simulink model "temp_ACGen_DCLink"  (R2013b)
settings: Solver=ode3  StartTime=0.0  StopTime=0.7  FixedStep=Ts  RelTol=1e-3
PreLoadFcn:
  | warning off Simulink:Commands:LoadMdlParameterizedLink
  | Ts=1e-5;
PostLoadFcn:
  | warning off Simulink:Commands:LoadMdlParameterizedLink
  | warning off Simulink:Engine:UsingDiscreteSolver
undefined symbols (not defined in the file or in its folder): D1, Delta
libraries: powerlib x21, powerlib_extras x5, Generator_Lib x1, simulink x1
Description:
  | Copyright 2013 The MathWorks, Inc.
settings Model: Creator=smiller  LastModifiedBy=smiller
settings DebuggingCC: StateNameClashWarn=warning

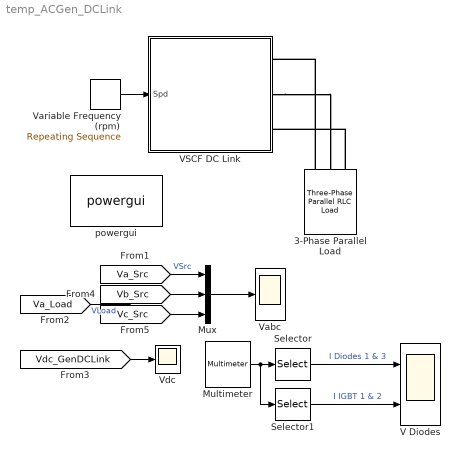
== system temp_ACGen_DCLink ==
  3-Phase Parallel Load : powerlib/Elements/Three-Phase Parallel RLC Load  LConnTagsString=A|B|C  Configuration=Y (grounded)  NominalVoltage=200  NominalFrequency=400  ActivePower=50e3  InductivePower=0  CapacitivePower=0  Measurements=None  LoadType=constant Z
  Multimeter : powerlib/Measurements/Multimeter  Tag=PoWeRsYsTeMmEaSuReMeNt  PhasorSimulation=off  OutputType=Magnitude  sel=[1 3 7 8]  L=12  Gain=[1 1 1 1]  yselected="{'Isw1: VSCF DC Link/Rect and Inv/Rectifier','Isw3: VSCF DC Link/Rect and Inv/Rectifier','Isw1: VSCF DC Link/Rect and Inv/PWM  IGBT Inverter','Isw2: VSCF DC Link/Rect and Inv/PWM  IGBT Inverter'};"  PSBOutputType=1  PSBequivalent=0  AxesSetting=[0,0.1,-100,100]  Display=0  SavedBlockNames=-11
      settings: AttributesFormatString=\n
  Mux : Mux  Inputs=3
  Selector : Selector  InputPortWidth=4  IndexOptions=Index vector (dialog)  Indices=[1 2]  OutputSizes=1
  Selector1 : Selector  InputPortWidth=4  IndexOptions=Index vector (dialog)  Indices=[3 4]  OutputSizes=1
  V Diodes : Scope  NumInputPorts=2
      settings: TimeRange=0.005  YMin=-10~-205  YMax=100~205
  VSCF DC Link : Subsystem
      mask Display:
      | image(imread('Gen_VSCF_DCLink_IMAGE.JPG','jpg'))
      | port_label('RConn',1,'A');
      | port_label('RConn',2,'B');
      | port_label('RConn',3,'C');
      | port_label('Input',1,'Spd');
  Vabc : Scope
      settings: TimeRange=0.0025  YMin=-200  YMax=200
  Variable Frequency (rpm) : simulink/Sources/Repeating Sequence  rep_seq_t=[0 1 2 3 4 5 6 7]/10  rep_seq_y=[1 1 0.9 0.95 0.8 0.96 1 1]*12000
  Vdc : Scope
      settings: TimeRange=0.0025  YMin=780  YMax=790  SaveName=ScopeData2
  powergui : powerlib/powergui  Priority=2  SimulationMode=Discrete  SolverType=Tustin  SampleTime=Ts  frequency=60  SPID=off  DisableSnubberDevices=off  DisableRonSwitches=off  DisableVfSwitches=off  SwTol=0  Interpol=off  DisplayEquations=off  frequencyindice=0  Pbase=100e6  ErrMax=1e-4  Iterations=50  UnitsV=kV  UnitsW=MW  FunctionMessages=off  echomessages=off  HookPort=off  EnableUseOfTLC=off  x0status=blocks  RestoreLinks=warning  ResistiveCurrentMeasurement=off  Frange=[0:2:500]  Ylog=off  Xlog=on  ShowGrid=off  save=off  variable=ZData  structure=psbbridges_str  ZoomFFT=on  StartTime=0.1-2/50  cycles=2  DisplayStyle=off  fundamental=50  FreqAxis=off  MaxFrequency=7000  frequencyindicesteady=1  RmsSteady=1  display=off  Ts=0  methode=off
  wires:
  Variable Frequency (rpm)/1 -> VSCF DC Link/1(Spd)
  [Va_Src] -> Mux/1  "VSrc"
  [Va_Load] -> ?  "VLoad"
  Selector/1 -> V Diodes/1  "I Diodes 1 & 3"
  Selector1/1 -> V Diodes/2  "I IGBT 1 & 2"
  Multimeter/1 -> Selector/1, Selector1/1
  [Vdc_GenDCLink] -> Vdc/1
  Mux/1 -> Vabc/1
  [Vb_Src] -> Mux/2
  [Vc_Src] -> Mux/3
  connections:
  3-Phase Parallel Load/LConn3 -- VSCF DC Link/RConn3
  3-Phase Parallel Load/LConn1 -- VSCF DC Link/RConn1
  VSCF DC Link/RConn2 -- 3-Phase Parallel Load/LConn2

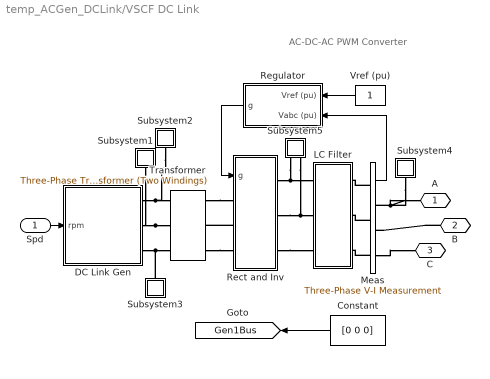
== system temp_ACGen_DCLink/VSCF DC Link ==
  note: AC-DC-AC PWM Converter
  Spd : Inport
  Constant : Constant  Value=[0 0 0]
  DC Link Gen : Subsystem  BlockChoice=Ideal
      settings: AttributesFormatString=%<BlockChoice>  TemplateBlock=Generator_Lib/DC Gen/DC Link Gen  MemberBlocks=Ideal,Sync Mach
  LC Filter : Subsystem
  Meas : powerlib/Measurements/Three-Phase V-I Measurement  VoltageMeasurement=phase-to-ground  SetLabelV=off  LabelV=V1  Vpu=on  VpuLL=off  CurrentMeasurement=no  SetLabelI=off  LabelI=I1  Ipu=off  Pbase=1e3  Vbase=200  OutputType=Magnitude  PhasorSimulation=off  PSBequivalent=0
  Rect and Inv : Subsystem
  Regulator : Subsystem
  Subsystem1 : Subsystem
      mask Display: disp('S')
  Subsystem2 : Subsystem
      mask Display: disp('S')
  Subsystem3 : Subsystem
      mask Display: disp('S')
  Subsystem4 : Subsystem
      mask Display: disp('S')
  Subsystem5 : Subsystem
      mask Display: disp('S')
  Transformer : powerlib/Elements/Three-Phase Transformer (Two Windings)  Winding1Connection=Yg  UNITS=pu  NominalPower=[ 50e3 , 800 ]  Winding1=[ 200 , 0.004 , 0.02 ]  Winding2Connection=Delta (D1)  Winding2=[ 600 , 0.004 , 0.02 ]  SetSaturation=off  Rm=200  Lm=200  Saturation="[ 0,0  ;  0.005,1.2  ;  1.0,1.4 ]"  Hysteresis=off  DataFile='hysteresis'  SetInitialFlux=off  InitialFluxes=[ 0.8 , -0.8 , 0.7 ]  Measurements=None  MoreParameters=off  BreakLoop=off  DataType=off  TransfoNumber=0
  "Vref (pu) " : Constant
  A : PMIOPort  Port=1  Side=Right
  B : PMIOPort  Port=2  Side=Right
  C : PMIOPort  Port=3  Side=Right
  tag scope: Gen1Bus=global
  wires:
  Constant/1 -> [Gen1Bus]
  Spd/1 -> DC Link Gen/1(rpm)
  Regulator/1(g) -> Rect and Inv/1(g)
  Meas/1 -> Regulator/2(Vabc (pu))
  "Vref (pu) "/1 -> Regulator/1(Vref (pu))
  connections:
  Rect and Inv/RConn3 -- LC Filter/LConn3
  Transformer/RConn3 -- Rect and Inv/LConn3
  Rect and Inv/LConn2 -- Transformer/RConn2
  DC Link Gen/RConn3 -- Subsystem3/LConn1 -- Transformer/LConn3
  Transformer/RConn1 -- Rect and Inv/LConn1
  Meas/LConn3 -- LC Filter/RConn3
  Meas/RConn3 -- C/RConn1
  Meas/LConn2 -- LC Filter/RConn2
  DC Link Gen/RConn2 -- Subsystem1/LConn1 -- Transformer/LConn2
  Meas/LConn1 -- LC Filter/RConn1
  B/RConn1 -- Meas/RConn2
  Rect and Inv/RConn1 -- Subsystem5/LConn1 -- LC Filter/LConn1
  Subsystem5/LConn2 -- Rect and Inv/RConn2 -- LC Filter/LConn2
  Subsystem2/LConn1 -- DC Link Gen/RConn1 -- Transformer/LConn1
  Meas/RConn1 -- A/RConn1 -- Subsystem4/LConn1

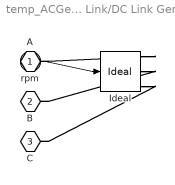
== system temp_ACGen_DCLink/VSCF DC Link/DC Link Gen ==
  rpm : Inport
  Ideal : Generator_Lib/DC Gen/Ideal  SystemSampleTime=-1
  A : PMIOPort  Port=1  Side=Right
  B : PMIOPort  Port=2  Side=Right
  C : PMIOPort  Port=3  Side=Right
  wires:
  rpm/1 -> Ideal/1
  connections:
  Ideal/RConn1 -- A/RConn1
  Ideal/RConn2 -- B/RConn1
  Ideal/RConn3 -- C/RConn1

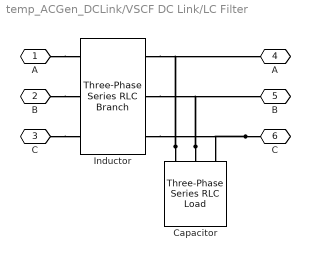
== system temp_ACGen_DCLink/VSCF DC Link/LC Filter ==
  Capacitor : powerlib/Elements/Three-Phase Series RLC Load  LConnTagsString=A|B|C  Configuration=Y (grounded)  NominalVoltage=200  NominalFrequency=400  ActivePower=0  InductivePower=0  CapacitivePower=3e3  Measurements=None  LoadType=constant Z
  Inductor : powerlib/Elements/Three-Phase Series RLC Branch  LConnTagsString=A|B|C  RConnTagsString=A|B|C  BranchType=L  Resistance=0  Inductance=2e-3*0.43  Capacitance=inf  Measurements=None
  A : PMIOPort  Port=1  Side=Left
  B : PMIOPort  Port=2  Side=Left
  C : PMIOPort  Port=3  Side=Left
  "A " : PMIOPort  Port=4  Side=Right
  "B " : PMIOPort  Port=5  Side=Right
  "C " : PMIOPort  Port=6  Side=Right
  connections:
  "C "/RConn1 -- Capacitor/LConn3 -- Inductor/RConn3
  Capacitor/LConn2 -- "B "/RConn1 -- Inductor/RConn2
  Capacitor/LConn1 -- "A "/RConn1 -- Inductor/RConn1
  C/RConn1 -- Inductor/LConn3
  A/RConn1 -- Inductor/LConn1
  B/RConn1 -- Inductor/LConn2

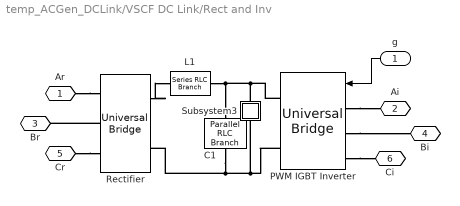
== system temp_ACGen_DCLink/VSCF DC Link/Rect and Inv ==
  g : Inport
  C1 : powerlib/Elements/Parallel RLC Branch  LConnTagsString=a  RConnTagsString=__new0  BranchType=C  Resistance=inf  Inductance=inf  SetiL0=off  InitialCurrent=0  Capacitance=5000e-06  Setx0=on  InitialVoltage=797  Measurements=None
  L1 : powerlib/Elements/Series RLC Branch  LConnTagsString=__new0  RConnTagsString=__new0  BranchType=L  Resistance=1.0  Inductance=200e-6  SetiL0=off  InitialCurrent=0  Capacitance=1.0  Setx0=off  InitialVoltage=0  Measurements=None
  PWM IGBT Inverter : powerlib/Power Electronics/Universal Bridge  Arms=3  SnubberResistance=5000  SnubberCapacitance=inf  Device=IGBT / Diodes  Ron=1e-3  Lon=0  ForwardVoltages="[  0.0  0.0  ]"  ForwardVoltage=.8  GTOparameters=[ 1e-6 ,1e-6 ]  IGBTparameters=[ 1e-6 , 2e-6 ]  Measurements=Device currents  Measurements_2=None  converterType=Rectifier
  Rectifier : powerlib/Power Electronics/Universal Bridge  Arms=3  SnubberResistance=100  SnubberCapacitance=0.1e-6  Device=Diodes  Ron=1e-3  Lon=0  ForwardVoltages="[  0.8  0.8  ]"  ForwardVoltage=.8  GTOparameters=[ 10e-6 , 20e-6 ]  IGBTparameters=[ 1e-6 , 2e-6 ]  Measurements=Device currents  Measurements_2=None  converterType=Rectifier
  Subsystem3 : Subsystem
      mask Display: disp('S')
  Ar : PMIOPort  Port=1  Side=Left
  Ai : PMIOPort  Port=2  Side=Right
  Br : PMIOPort  Port=3  Side=Left
  Bi : PMIOPort  Port=4  Side=Right
  Cr : PMIOPort  Port=5  Side=Left
  Ci : PMIOPort  Port=6  Side=Right
  wires:
  g/1 -> PWM IGBT Inverter/1
  connections:
  PWM IGBT Inverter/LConn1 -- Ai/RConn1
  PWM IGBT Inverter/LConn2 -- Bi/RConn1
  Rectifier/LConn2 -- Br/RConn1
  Ar/RConn1 -- Rectifier/LConn1
  Cr/RConn1 -- Rectifier/LConn3
  Subsystem3/LConn1 -- PWM IGBT Inverter/RConn1 -- C1/LConn1 -- L1/RConn1
  Subsystem3/RConn1 -- Rectifier/RConn2 -- C1/RConn1 -- PWM IGBT Inverter/RConn2
  Rectifier/RConn1 -- L1/LConn1
  PWM IGBT Inverter/LConn3 -- Ci/RConn1

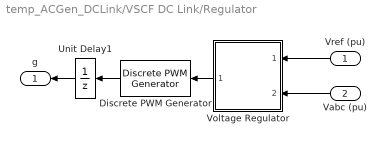
== system temp_ACGen_DCLink/VSCF DC Link/Regulator ==
  Vref (pu) : Inport
  Vabc (pu) : Inport  Port=2
  Discrete PWM Generator : powerlib_extras/Discrete  Control Blocks/Discrete PWM Generator  GeneratorMode="3-arm  bridge (6 pulses)"  Fc=10000  Ts=Ts  Internal=off  mIndex=0.4  Freq=60  Phase=0
  Unit Delay1 : UnitDelay  SampleTime=Ts
  Voltage Regulator : Subsystem  mask(Voltage Regulator){Kp=0.4, Ki=500, Ts=Ts}
      mask prompts: Kp "Proportional gain  Kp:"; Ki "Integral gain Ki:"; Ts "Sample time (s) :"
  g : Outport
  wires:
  Unit Delay1/1 -> g/1
  Discrete PWM Generator/1 -> Unit Delay1/1
  Vref (pu)/1 -> Voltage Regulator/1(Vd_ref (pu))
  Vabc (pu)/1 -> Voltage Regulator/2(Vabc (pu))
  Voltage Regulator/1(Vabc_inv) -> Discrete PWM Generator/1

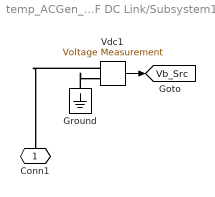
== system temp_ACGen_DCLink/VSCF DC Link/Subsystem1 ==
  Ground : powerlib/Elements/Ground  LConnTagsString=a
  Vdc1 : powerlib/Measurements/Voltage Measurement  Tag=PoWeRsYsTeMmEaSuReMeNt  PhasorSimulation=off  OutputType=Magnitude  PSBequivalent=0
  Conn1 : PMIOPort  Port=1  Side=Left
  tag scope: Vb_Src=global
  wires:
  Vdc1/1 -> [Vb_Src]
  connections:
  Vdc1/LConn1 -- Conn1/RConn1
  Ground/LConn1 -- Vdc1/LConn2

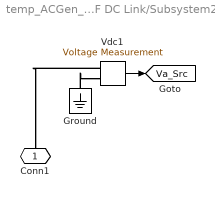
== system temp_ACGen_DCLink/VSCF DC Link/Subsystem2 ==
  Ground : powerlib/Elements/Ground  LConnTagsString=a
  Vdc1 : powerlib/Measurements/Voltage Measurement  Tag=PoWeRsYsTeMmEaSuReMeNt  PhasorSimulation=off  OutputType=Magnitude  PSBequivalent=0
  Conn1 : PMIOPort  Port=1  Side=Left
  tag scope: Va_Src=global
  wires:
  Vdc1/1 -> [Va_Src]
  connections:
  Ground/LConn1 -- Vdc1/LConn2
  Vdc1/LConn1 -- Conn1/RConn1

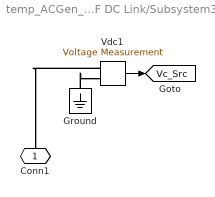
== system temp_ACGen_DCLink/VSCF DC Link/Subsystem3 ==
  Ground : powerlib/Elements/Ground  LConnTagsString=a
  Vdc1 : powerlib/Measurements/Voltage Measurement  Tag=PoWeRsYsTeMmEaSuReMeNt  PhasorSimulation=off  OutputType=Magnitude  PSBequivalent=0
  Conn1 : PMIOPort  Port=1  Side=Left
  tag scope: Vc_Src=global
  wires:
  Vdc1/1 -> [Vc_Src]
  connections:
  Vdc1/LConn1 -- Conn1/RConn1
  Ground/LConn1 -- Vdc1/LConn2

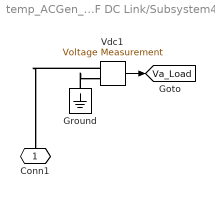
== system temp_ACGen_DCLink/VSCF DC Link/Subsystem4 ==
  Ground : powerlib/Elements/Ground  LConnTagsString=a
  Vdc1 : powerlib/Measurements/Voltage Measurement  Tag=PoWeRsYsTeMmEaSuReMeNt  PhasorSimulation=off  OutputType=Magnitude  PSBequivalent=0
  Conn1 : PMIOPort  Port=1  Side=Left
  tag scope: Va_Load=global
  wires:
  Vdc1/1 -> [Va_Load]
  connections:
  Vdc1/LConn1 -- Conn1/RConn1
  Ground/LConn1 -- Vdc1/LConn2

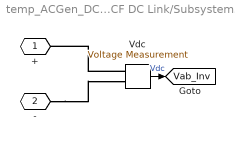
== system temp_ACGen_DCLink/VSCF DC Link/Subsystem5 ==
  Vdc : powerlib/Measurements/Voltage Measurement  Tag=PoWeRsYsTeMmEaSuReMeNt  PhasorSimulation=off  OutputType=Magnitude  PSBequivalent=0
  + : PMIOPort  Port=1  Side=Left
  - : PMIOPort  Port=2  Side=Left
  tag scope: Vab_Inv=global
  wires:
  Vdc/1 -> [Vab_Inv]  "Vdc"
  connections:
  Vdc/LConn1 -- +/RConn1
  -/RConn1 -- Vdc/LConn2

== system temp_ACGen_DCLink/VSCF DC Link/Rect and Inv/Subsystem3 ==
  Vdc : powerlib/Measurements/Voltage Measurement  Tag=PoWeRsYsTeMmEaSuReMeNt  PhasorSimulation=off  OutputType=Magnitude  PSBequivalent=0
  + : PMIOPort  Port=1  Side=Left
  - : PMIOPort  Port=2  Side=Right
  tag scope: Vdc_GenDCLink=global
  wires:
  Vdc/1 -> [Vdc_GenDCLink]  "Vdc"
  connections:
  -/RConn1 -- Vdc/LConn2
  Vdc/LConn1 -- +/RConn1

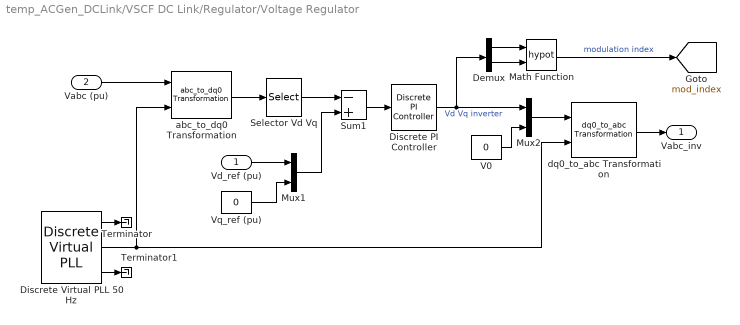
== system temp_ACGen_DCLink/VSCF DC Link/Regulator/Voltage Regulator ==
  Vd_ref (pu) : Inport
  Vabc (pu) : Inport  Port=2
  Demux : Demux  Outputs=2
  Discrete PI Controller : powerlib_extras/Discrete  Control Blocks/Discrete PI Controller  Kp=Kp  Ki=Ki  Par_Limits=[1 -1]  Init=0  Ts=Ts
  Discrete Virtual PLL 50 Hz : powerlib_extras/Discrete  Control Blocks/Discrete Virtual PLL  Freq=400  Phase=0  Ts=Ts
  Math Function : Math  Operator=hypot  SaturateOnIntegerOverflow=on
  Mux1 : Mux  Inputs=2
  Mux2 : Mux  Inputs=2
  Selector Vd Vq : Selector  InputPortWidth=3  IndexOptions=Index vector (dialog)  Indices=[1 2]  OutputSizes=1
  Sum1 : Sum  Inputs=-+  SaturateOnIntegerOverflow=on  InputSameDT=on  OutDataTypeStr=Inherit: Same as first input
  Terminator : Terminator
  Terminator1 : Terminator
  V0 : Constant  Value=0
  Vq_ref (pu) : Constant  Value=0
  abc_to_dq0 Transformation : powerlib_extras/Measurements/abc_to_dq0 Transformation
  dq0_to_abc Transformation : powerlib_extras/Measurements/dq0_to_abc Transformation
  Vabc_inv : Outport
  tag scope: mod_index=global
  wires:
  Math Function/1 -> [mod_index]  "modulation index"
  Demux/2 -> Math Function/2
  Demux/1 -> Math Function/1
  Discrete PI Controller/1 -> Mux2/1, Demux/1  "Vd Vq inverter"
  Discrete Virtual PLL 50 Hz/3 -> Terminator1/1
  Discrete Virtual PLL 50 Hz/1 -> Terminator/1
  Mux1/1 -> Sum1/2
  Vq_ref (pu)/1 -> Mux1/2
  Vd_ref (pu)/1 -> Mux1/1
  Discrete Virtual PLL 50 Hz/2 -> dq0_to_abc Transformation/2, abc_to_dq0 Transformation/2
  dq0_to_abc Transformation/1 -> Vabc_inv/1
  V0/1 -> Mux2/2
  Mux2/1 -> dq0_to_abc Transformation/1
  Sum1/1 -> Discrete PI Controller/1
  Selector Vd Vq/1 -> Sum1/1
  Vabc (pu)/1 -> abc_to_dq0 Transformation/1
  abc_to_dq0 Transformation/1 -> Selector Vd Vq/1
